simulink model "LQR_discrete"  (Simulink 10.3)
settings: Solver=ode45  StartTime=0.0  StopTime=tsim  RelTol=1e-3  EnableMultiTasking=on
values from neighbouring files (symbols this model uses):
  A = [-1.2822 0 0.98 0; 0 0 1 0; -5.4293 0 -1.8366 0; -128.2 128.2 0 0]    [Razzo27.m]
  B = [-0.3 0 -17 0]'    [Razzo27.m]
  C = [0 1 0 0; 0 0 0 1; -128.2 128.2 0 0]    [Razzo27.m]
  C_states = eye(4)    [Razzo27.m]
  D_states = [0; 0; 0; 0]    [Razzo27.m]
  Klqr_LQ = Klqr4    [Razzo27.m]
  sat_max = deg2rad(15)    [Razzo27.m]
  sat_min = deg2rad(-15)    [Razzo27.m]
  sysd = c2d(sys,Ts)    [Razzo27.m]
  Ts = 0.5*(T_taglio/2)    [Razzo27.m]
  x0 = [deg2rad(0) deg2rad(-15) 0 200]    [Razzo27.m]
  x_ref = [0 0 0 0]'    [Razzo27.m]
undefined symbols (not defined in the file or in its folder): Klqr_d
settings Model: Creator=Administrator  LastModifiedBy=dadel  MultithreadedSim=on
settings DataIOCC: LimitDataPoints=on
settings OptimizationCC: InitFltsAndDblsToZero=on
settings DebuggingCC: SolverPrmCheckMsg=warning
settings ConfigComp: CovSFcnEnable=off

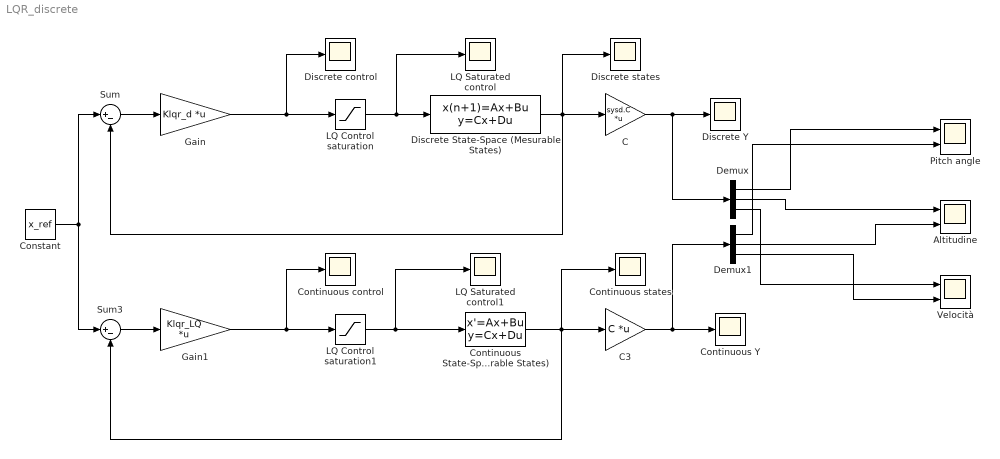
== system LQR_discrete ==
  Altitudine : Scope  NumInputPorts=2
  C : Gain  Gain=sysd.C  Multiplication=Matrix(K*u)
  C3 : Gain  Gain=C  Multiplication=Matrix(K*u)
  Constant : Constant  Value=x_ref
  Continuous State-Space (Mesurable States) : StateSpace  A=A  B=B  C=C_states  D=D_states  InitialCondition=x0
  Continuous Y : Scope
  Continuous control : Scope
  Continuous states : Scope
  Demux : Demux  Outputs=3
  Demux1 : Demux  Outputs=3
  Discrete State-Space (Mesurable States) : DiscreteStateSpace  A=sysd.A  B=sysd.B  C=C_states  D=D_states  InitialCondition=x0  SampleTime=Ts
  Discrete Y : Scope
  Discrete control : Scope
  Discrete states : Scope
  Gain : Gain  Gain=Klqr_d  Multiplication=Matrix(K*u)
  Gain1 : Gain  Gain=Klqr_LQ  Multiplication=Matrix(K*u)
  LQ Control saturation : Saturate  UpperLimit=sat_max  LowerLimit=sat_min
  LQ Control saturation1 : Saturate  UpperLimit=sat_max  LowerLimit=sat_min
  LQ Saturated control : Scope
  LQ Saturated control1 : Scope
  Pitch angle : Scope  NumInputPorts=2
  Sum : Sum  Inputs=|+-
  Sum3 : Sum  Inputs=|+-
  Velocità : Scope  NumInputPorts=2
  wires:
  Gain/1 -> LQ Control saturation/1, Discrete control/1
  Sum/1 -> Gain/1
  Discrete State-Space (Mesurable States)/1 -> C/1, Discrete states/1, Sum/2
  C/1 -> Demux/1, Discrete Y/1
  Gain1/1 -> LQ Control saturation1/1, Continuous control/1
  Continuous State-Space (Mesurable States)/1 -> Continuous states/1, C3/1, Sum3/2
  C3/1 -> Demux1/1, Continuous Y/1
  Sum3/1 -> Gain1/1
  Demux/1 -> Pitch angle/1
  Demux1/1 -> Pitch angle/2
  Demux/2 -> Altitudine/1
  Demux1/2 -> Altitudine/2
  Demux/3 -> Velocità/1
  Demux1/3 -> Velocità/2
  Constant/1 -> Sum3/1, Sum/1
  LQ Control saturation/1 -> LQ Saturated control/1, Discrete State-Space (Mesurable States)/1
  LQ Control saturation1/1 -> LQ Saturated control1/1, Continuous State-Space (Mesurable States)/1
